simulink model "PID_controldesign"  (R2024b)
settings: Solver=VariableStepAuto  StartTime=0.0  StopTime=10.0  RelTol=1e-3
values from neighbouring files (symbols this model uses):
  current2Torque = mot.Kt    [simulation.m]
  denDriv = [Tdrv 1]    [simulation.m]
  denElect = [mot.L Req]    [simulation.m]
  denMech = [J_eq B_eq]    [simulation.m]
  Kd = Kp * Td    [PID_SCRIPT.m]    (also in PID_controller.m; simulation.m)
  Ki = Kp / Ti    [PID_SCRIPT.m]    (also in PID_controller.m; simulation.m)
  Kp = delta_K*cos(delta_Phi)    [PID_SCRIPT.m]    (also in PID_controller.m; simulation.m = delta_k * cosd(delta_phi))
  Kw = 1/Tw    (= 5.88235294118)    [PID_SCRIPT.m]    (also in PID_controller.m)
  numDriv = [kdrv]    [simulation.m]
  numElect = [1]    [simulation.m]
  numMech = [1]    [simulation.m]
  speed2Voltage = mot.Ke    [simulation.m]
  Tau = 9.4e-3    (= 0.0094)    [StateSpaceScript.m]
  Tl = 1/(10*omega_gc)    [PID_SCRIPT.m]    (also in PID_controller.m)
undefined symbols (not defined in the file or in its folder): daq, denBeam, drv, gbox, kappa, numBeam, rads2rpm, sens
settings Model: Creator=Davide Pillon  LastModifiedBy=Davide Pillon

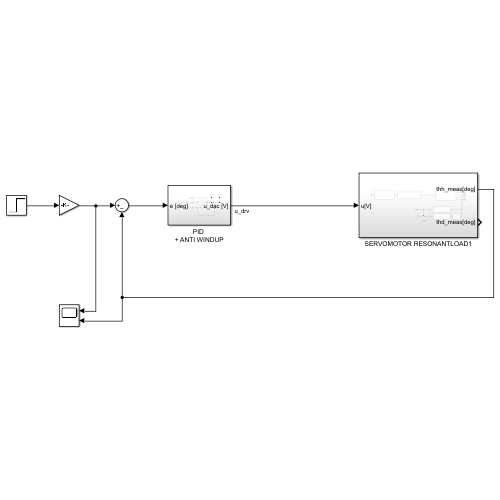
[thumbnail: Simulink's stored preview of the top-level diagram]
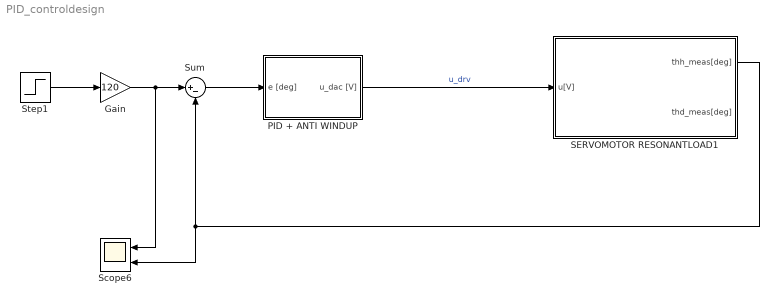
== system PID_controldesign ==
  Gain : Gain  Gain=120
  PID + ANTI WINDUP : Subsystem
  SERVOMOTOR RESONANTLOAD1 : Subsystem
  Scope6 : Scope  NumInputPorts=2
  Step1 : Step  SampleTime=0
  Sum : Sum  Inputs=|+-
  wires:
  Step1/1 -> Gain/1
  PID + ANTI WINDUP/1(u_dac [V]) -> SERVOMOTOR RESONANTLOAD1/1(u[V])  "u_drv"
  Gain/1 -> Scope6/1, Sum/1
  SERVOMOTOR RESONANTLOAD1/1(thh_meas[deg]) -> Sum/2, Scope6/2
  Sum/1 -> PID + ANTI WINDUP/1(e [deg])

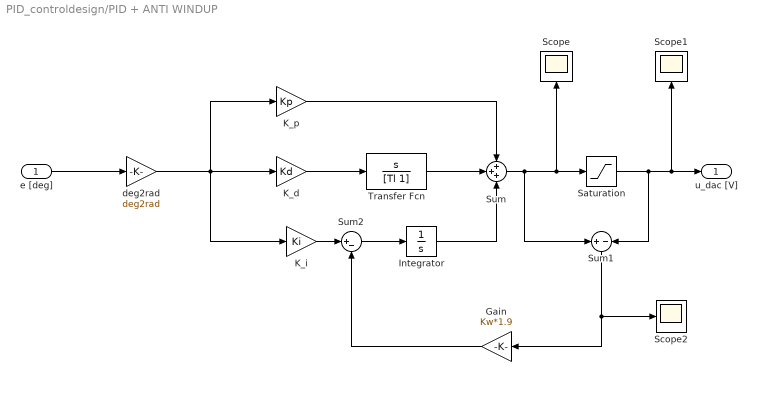
== system PID_controldesign/PID + ANTI WINDUP ==
  e [deg] : Inport
  Gain : Gain  Gain=Kw*1.9
  Integrator : Integrator
  K_d : Gain  Gain=Kd
  K_i : Gain  Gain=Ki
  K_p : Gain  Gain=Kp
  Saturation : Saturate  UpperLimit=10  LowerLimit=-10
  Scope : Scope
  Scope1 : Scope
  Scope2 : Scope
  Sum : Sum  Inputs=+++
  Sum1 : Sum  Inputs=+-
  Sum2 : Sum  Inputs=|+-
  Transfer Fcn : TransferFcn  Numerator=[1 0]  Denominator=[Tl 1]
  deg2rad : Gain  Gain=deg2rad
  u_dac [V] : Outport
  wires:
  e [deg]/1 -> deg2rad/1
  Transfer Fcn/1 -> Sum/2
  Integrator/1 -> Sum/3
  deg2rad/1 -> K_i/1, K_d/1, K_p/1
  K_p/1 -> Sum/1
  K_i/1 -> Sum2/1
  Sum2/1 -> Integrator/1
  K_d/1 -> Transfer Fcn/1
  Sum1/1 -> Scope2/1, Gain/1
  Sum/1 -> Sum1/1, Saturation/1, Scope/1
  Saturation/1 -> Scope1/1, u_dac [V]/1, Sum1/2
  Gain/1 -> Sum2/2

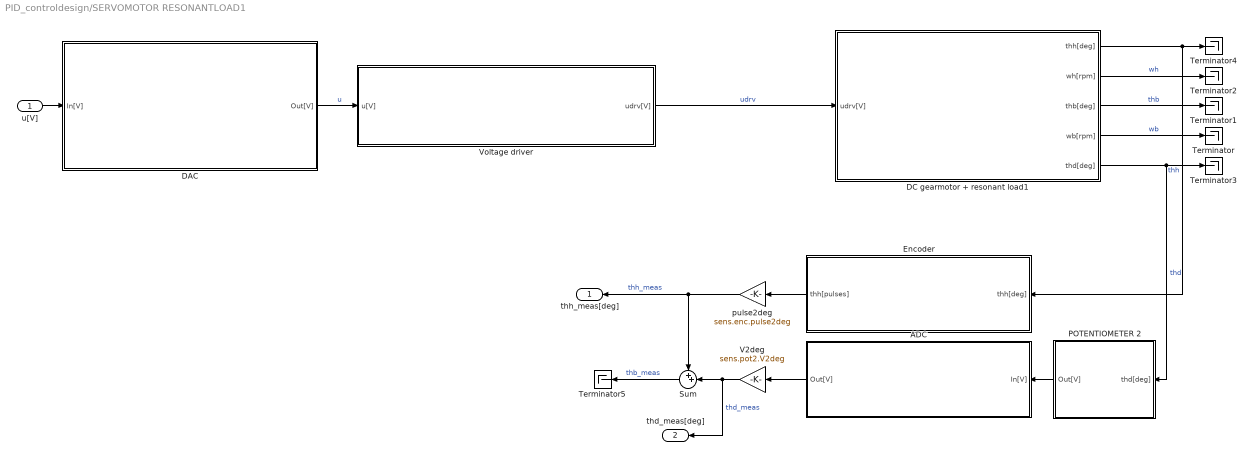
== system PID_controldesign/SERVOMOTOR RESONANTLOAD1 ==
  u[V] : Inport
  ADC : Subsystem
  DAC : Subsystem
  DC gearmotor + resonant load1 : Subsystem
  Encoder : Subsystem
  POTENTIOMETER 2 : Subsystem
  Sum : Sum  Inputs=++|
  Terminator{,1..5} (6 alike) : Terminator
  V2deg : Gain  Gain=sens.pot2.V2deg
  Voltage driver : Subsystem
  pulse2deg : Gain  Gain=sens.enc.pulse2deg
  thh_meas[deg] : Outport
  thd_meas[deg] : Outport  Port=2
  wires:
  DC gearmotor + resonant load1/3(thb[deg]) -> Terminator1/1  "thb"
  DC gearmotor + resonant load1/2(wh[rpm]) -> Terminator2/1  "wh"
  DAC/1(Out[V]) -> Voltage driver/1(u[V])  "u"
  Sum/1 -> Terminator5/1  "thb_meas"
  ADC/1(Out[V]) -> V2deg/1
  DC gearmotor + resonant load1/1(thh[deg]) -> Encoder/1(thh[deg]), Terminator4/1  "thh"
  pulse2deg/1 -> thh_meas[deg]/1, Sum/1  "thh_meas"
  V2deg/1 -> thd_meas[deg]/1, Sum/2  "thd_meas"
  Encoder/1(thh[pulses]) -> pulse2deg/1
  POTENTIOMETER 2/1(Out[V]) -> ADC/1(In[V])
  Voltage driver/1(udrv[V]) -> DC gearmotor + resonant load1/1(udrv[V])  "udrv"
  u[V]/1 -> DAC/1(In[V])
  DC gearmotor + resonant load1/4(wb[rpm]) -> Terminator/1  "wb"
  DC gearmotor + resonant load1/5(thd[deg]) -> POTENTIOMETER 2/1(thd[deg]), Terminator3/1  "thd"

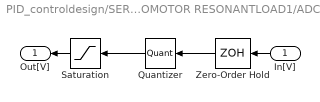
== system PID_controldesign/SERVOMOTOR RESONANTLOAD1/ADC ==
  In[V] : Inport
  Quantizer : Quantizer  QuantizationInterval=daq.adc.q
  Saturation : Saturate  UpperLimit=daq.adc.fs  LowerLimit=-daq.adc.fs
  Zero-Order Hold : ZeroOrderHold  SampleTime=daq.adc.ts
  Out[V] : Outport
  wires:
  Saturation/1 -> Out[V]/1
  In[V]/1 -> Zero-Order Hold/1
  Zero-Order Hold/1 -> Quantizer/1
  Quantizer/1 -> Saturation/1

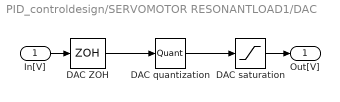
== system PID_controldesign/SERVOMOTOR RESONANTLOAD1/DAC ==
  In[V] : Inport
  DAC ZOH : ZeroOrderHold  SampleTime=daq.dac.ts
  DAC quantization : Quantizer  QuantizationInterval=daq.dac.q
  DAC saturation : Saturate  UpperLimit=daq.dac.fs  LowerLimit=-daq.dac.fs
  Out[V] : Outport
  wires:
  DAC saturation/1 -> Out[V]/1
  In[V]/1 -> DAC ZOH/1
  DAC ZOH/1 -> DAC quantization/1
  DAC quantization/1 -> DAC saturation/1

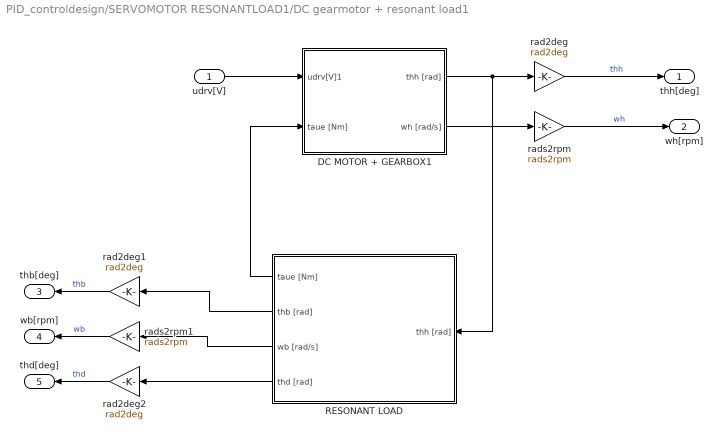
== system PID_controldesign/SERVOMOTOR RESONANTLOAD1/DC gearmotor + resonant load1 ==
  udrv[V] : Inport
  DC MOTOR + GEARBOX1 : Subsystem
  RESONANT LOAD : Subsystem
  rad2deg : Gain  Gain=rad2deg
  rad2deg1 : Gain  Gain=rad2deg
  rad2deg2 : Gain  Gain=rad2deg
  rads2rpm : Gain  Gain=rads2rpm
  rads2rpm1 : Gain  Gain=rads2rpm
  thh[deg] : Outport
  wh[rpm] : Outport  Port=2
  thb[deg] : Outport  Port=3
  wb[rpm] : Outport  Port=4
  thd[deg] : Outport  Port=5
  wires:
  rad2deg/1 -> thh[deg]/1  "thh"
  rad2deg2/1 -> thd[deg]/1  "thd"
  udrv[V]/1 -> DC MOTOR + GEARBOX1/1(udrv[V]1)
  RESONANT LOAD/4(thd [rad]) -> rad2deg2/1
  RESONANT LOAD/2(thb [rad]) -> rad2deg1/1
  RESONANT LOAD/3(wb [rad/s]) -> rads2rpm1/1
  DC MOTOR + GEARBOX1/2(wh [rad/s]) -> rads2rpm/1
  rad2deg1/1 -> thb[deg]/1  "thb"
  DC MOTOR + GEARBOX1/1(thh [rad]) -> RESONANT LOAD/1(thh [rad]), rad2deg/1
  rads2rpm1/1 -> wb[rpm]/1  "wb"
  RESONANT LOAD/1(taue [Nm]) -> DC MOTOR + GEARBOX1/2(taue [Nm])
  rads2rpm/1 -> wh[rpm]/1  "wh"

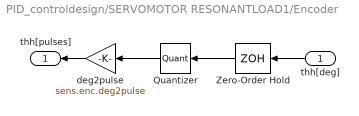
== system PID_controldesign/SERVOMOTOR RESONANTLOAD1/Encoder ==
  thh[deg] : Inport
  Quantizer : Quantizer  QuantizationInterval=daq.adc.q
  Zero-Order Hold : ZeroOrderHold  SampleTime=daq.adc.ts
  deg2pulse : Gain  Gain=sens.enc.deg2pulse
  thh[pulses] : Outport
  wires:
  thh[deg]/1 -> Zero-Order Hold/1
  deg2pulse/1 -> thh[pulses]/1
  Quantizer/1 -> deg2pulse/1
  Zero-Order Hold/1 -> Quantizer/1

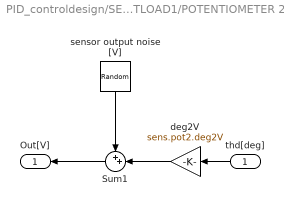
== system PID_controldesign/SERVOMOTOR RESONANTLOAD1/POTENTIOMETER 2 ==
  thd[deg] : Inport
  Sum1 : Sum  Inputs=++|
  deg2V : Gain  Gain=sens.pot2.deg2V
  sensor output noise [V] : RandomNumber  Variance=sens.pot2.noise.var  SampleTime=sens.pot2.Ts
  Out[V] : Outport
  wires:
  thd[deg]/1 -> deg2V/1
  deg2V/1 -> Sum1/2
  sensor output noise [V]/1 -> Sum1/1
  Sum1/1 -> Out[V]/1

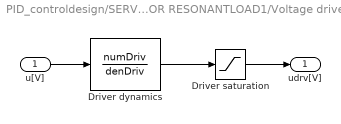
== system PID_controldesign/SERVOMOTOR RESONANTLOAD1/Voltage driver ==
  u[V] : Inport
  Driver dynamics : TransferFcn  Numerator=numDriv  Denominator=denDriv
  Driver saturation : Saturate  UpperLimit=drv.outmax  LowerLimit=-drv.outmax
  udrv[V] : Outport
  wires:
  u[V]/1 -> Driver dynamics/1
  Driver saturation/1 -> udrv[V]/1
  Driver dynamics/1 -> Driver saturation/1

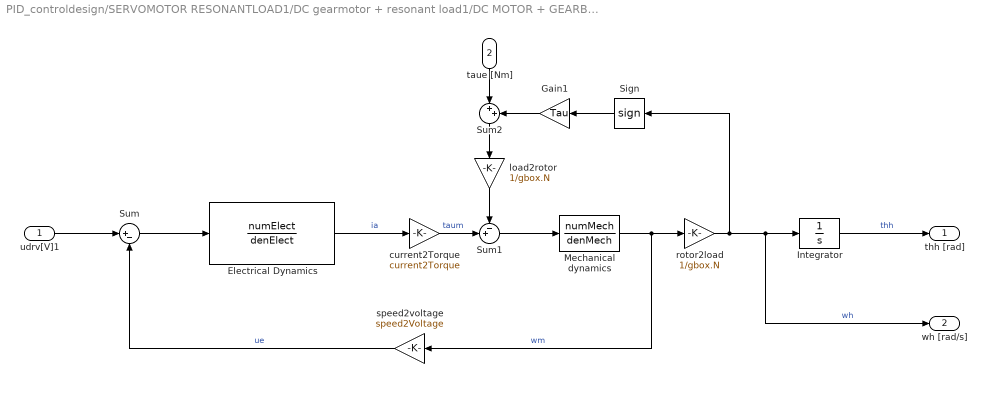
== system PID_controldesign/SERVOMOTOR RESONANTLOAD1/DC gearmotor + resonant load1/DC MOTOR + GEARBOX1 ==
  udrv[V]1 : Inport
  taue [Nm] : Inport  Port=2
  " Electrical Dynamics" : TransferFcn  Numerator=numElect  Denominator=denElect
  Gain1 : Gain  Gain=Tau
  Integrator : Integrator
  Mechanical dynamics : TransferFcn  Numerator=numMech  Denominator=denMech
  Sign : Signum  ZeroCross=off
  Sum : Sum  Inputs=|+-
  Sum1 : Sum  Inputs=-+|
  Sum2 : Sum  Inputs=|++
  current2Torque : Gain  Gain=current2Torque
  load2rotor : Gain  Gain=1/gbox.N
  rotor2load : Gain  Gain=1/gbox.N
  speed2voltage : Gain  Gain=speed2Voltage
  thh [rad] : Outport
  wh [rad/s] : Outport  Port=2
  wires:
  Integrator/1 -> thh [rad]/1  "thh"
  rotor2load/1 -> Sign/1, wh [rad/s]/1, Integrator/1  "wh"
  udrv[V]1/1 -> Sum/1
  Sum/1 -> " Electrical Dynamics"/1
  current2Torque/1 -> Sum1/2  "taum"
  Sign/1 -> Gain1/1
  Sum2/1 -> load2rotor/1
  speed2voltage/1 -> Sum/2  "ue"
  Gain1/1 -> Sum2/2
  " Electrical Dynamics"/1 -> current2Torque/1  "ia"
  Sum1/1 -> Mechanical dynamics/1
  taue [Nm]/1 -> Sum2/1
  load2rotor/1 -> Sum1/1
  Mechanical dynamics/1 -> speed2voltage/1, rotor2load/1  "wm"

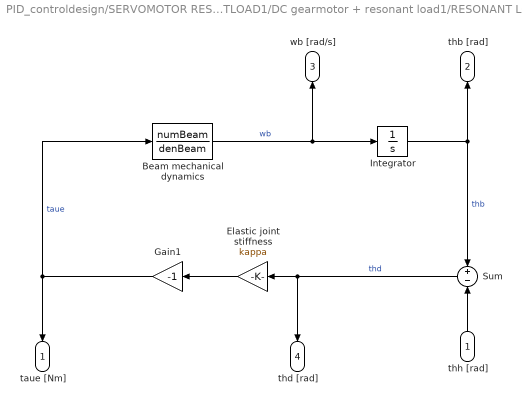
== system PID_controldesign/SERVOMOTOR RESONANTLOAD1/DC gearmotor + resonant load1/RESONANT LOAD ==
  thh [rad] : Inport
  Beam mechanical dynamics : TransferFcn  Numerator=numBeam  Denominator=denBeam
  Elastic joint stiffness : Gain  Gain=kappa
  Gain1 : Gain  Gain=-1
  Integrator : Integrator
  Sum : Sum  Inputs=+-
  taue [Nm] : Outport
  thb [rad] : Outport  Port=2
  wb [rad/s] : Outport  Port=3
  thd [rad] : Outport  Port=4
  wires:
  Integrator/1 -> thb [rad]/1, Sum/1  "thb"
  Beam mechanical dynamics/1 -> wb [rad/s]/1, Integrator/1  "wb"
  Elastic joint stiffness/1 -> Gain1/1
  Sum/1 -> thd [rad]/1, Elastic joint stiffness/1  "thd"
  Gain1/1 -> taue [Nm]/1, Beam mechanical dynamics/1  "taue"
  thh [rad]/1 -> Sum/2
